simulink model "TrafficLight"  (R2020a)
settings: Solver=FixedStepDiscrete  StartTime=0.0  StopTime=50  RelTol=1e-3
settings Model: Creator=yomna  LastModifiedBy=yomna
settings OptimizationCC: DefaultParameterBehavior=Inlined  EnhancedBackFolding=on  PassReuseOutputArgsAs=Individual arguments  ZeroExternalMemoryAtStartup=off  ZeroInternalMemoryAtStartup=off  OptimizeBlockOrder=speed  DifferentSizesBufferReuse=on  OptimizationCustomize=off  EfficientTunableParamExpr=on
settings DebuggingCC: UnderspecifiedInitializationDetection=Classic  MergeDetectMultiDrivingBlocksExec=none  ParameterTunabilityLossMsg=error
settings ModelReferenceCC: PropagateSignalLabelsOutOfModel=off
settings SFSimCC: MATLABDynamicMemAlloc=off
settings RTWCC: SystemTargetFile=ert.tlc  GenCodeOnly=on  TemplateMakefile=ert_default_tmf  GenerateReport=on  IncludeHyperlinkInReport=on  LaunchReport=on  GenerateTraceInfo=on  GenerateTraceReport=on  GenerateTraceReportSl=on  GenerateTraceReportSf=on  GenerateTraceReportEml=on
settings CodeAppCC: ForceParamTrailComments=on  IgnoreCustomStorageClasses=off  OperatorAnnotations=on  SimulinkDataObjDesc=on  SFDataObjDesc=on  InsertBlockDesc=on
settings ERTTargetCC: TargetLangStandard=C99 (ISO)  GenerateSampleERTMain=on  InlinedParameterPlacement=NonHierarchical  ERTCustomFileTemplate=example_file_process.tlc

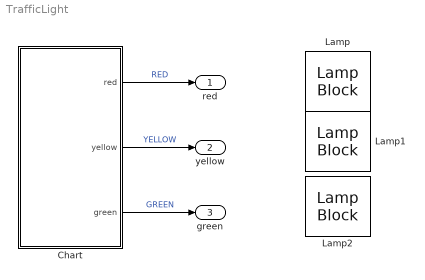
== system TrafficLight ==
  Chart : Stateflow chart  TreatAsAtomicUnit=on
  Lamp : LampBlock
  Lamp1 : LampBlock
  Lamp2 : LampBlock
  red : Outport
  yellow : Outport  Port=2
  green : Outport  Port=3
  wires:
  Chart/1(red) -> red/1  "RED"
  Chart/2(yellow) -> yellow/1  "YELLOW"
  Chart/3(green) -> green/1  "GREEN"

== stateflow chart TrafficLight/Chart ==
  state stop2
    en:
    red = uint8(1)
    yellow = uint8(0)
    green = uint8(0)
    du:
    red = uint8(0)
    yellow = uint8(1)
    green = uint8(0)
    ex:
    red = uint8(0)
    yellow = uint8(1)
    green = uint8(0)
  state stop
    en:
    red = uint8(0)
    yellow = uint8(0)
    green = uint8(0)
    du:
    red = uint8(1)
    yellow = uint8(0)
    green = uint8(0)
    ex:
    red = uint8(1)
    yellow = uint8(0)
    green = uint8(0)
  state stop1
    en:
    red = uint8(0)
    yellow = uint8(1)
    green = uint8(0)
    du:
    red = uint8(0)
    yellow = uint8(0)
    green = uint8(1)
    ex:
    red = uint8(0)
    yellow = uint8(0)
    green = uint8(1)
  (default) -> stop
  stop -> stop2 : after(3000,msec)
  stop2 -> stop1 : after(3000,msec)
  stop1 -> stop : after(3000,msec)
  data: red output uint8; yellow output uint8; green output uint8
